simulink library "sm_trackV_lib_chain_underc_i1u2l7"  (R2026a)
settings: Solver=VariableStepAuto
undefined symbols (not defined in the file): Excv, Left, P1, P2, P3, P4, P5, P6, P7, P8, P9, Right
libraries: sm_trackV_lib_chain_underc_elem x26, sm_lib x24, nesl_utility x20, fl_lib x4, sm_trackV_lib_frame_i1u2l7 x2
(part 2 of 2)

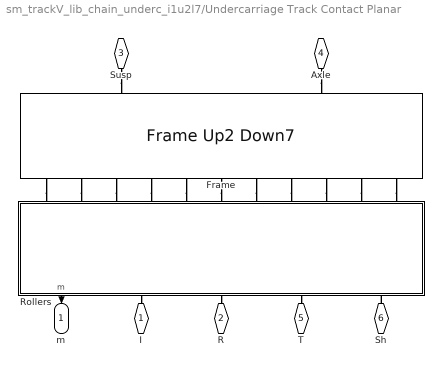
== system sm_trackV_lib_chain_underc_i1u2l7/Undercarriage Track Contact Planar ==
  Frame : sm_trackV_lib_frame_i1u2l7/Frame Up2 Down7  popup_leftOrRight=Right  roller_upper_x=roller_upper_x  roller_lower_x=roller_lower_x  idler_x=idler_x  axle_x=axle_x  roller_upper_y=roller_upper_y  roller_lower_y=roller_lower_y  idler_y=idler_y  axle_y=axle_y  frame_cg_offset=frame_cg_offset  frame_mass=frame_mass  frame_moi=frame_moi  frame_poi=frame_poi  frame_susp_offset=frame_susp_offset
  Rollers : Subsystem  mask(Rollers for Integration with Track Model){sprk_xc=sprk_xc, sprk_len=sprk_len, sprk_rho=sprk_rho, sprk_clr=sprk_clr, sprk_opc=sprk_opc, sprk_contact_geo_ptcld=sprk_contact_geo_ptcld, sprk_contact_geo_rad=sprk_contact_geo_rad, sprk_contact_geo_clr=sprk_contact_geo_clr, sprk_contact_geo_opc=sprk_contact_geo_opc, idler_rad=idler_rad, idler_len=idler_len, idler_rho=idler_rho, idler_clr=idler_clr, idler_opc=idler_opc, idler_contgeo_clr=idler_contgeo_clr, idler_contgeo_opc=idler_contgeo_opc, roller_upper_len=roller_upper_len, roller_upper_rad=roller_upper_rad, roller_upper_rho=roller_upper_rho, roller_upper_clr=roller_upper_clr, roller_upper_opc=roller_upper_opc, roller_upper_contgeo_clr=roller_upper_contgeo_clr, roller_upper_contgeo_opc=roller_upper_contgeo_opc, roller_lower_len=roller_lower_len, roller_lower_rad=roller_lower_rad, roller_lower_rho=roller_lower_rho, roller_lower_clr=roller_lower_clr, roller_lower_opc=roller_lower_opc, roller_lower_contgeo_clr=roller_lower_contgeo_clr, roller_lower_contgeo_opc=roller_lower_contgeo_opc, tensioner_cyl_rad=tensioner_cyl_rad, tensioner_cyl_len=tensioner_cyl_len, tensioner_cyl_rho=tensioner_cyl_rho, tensioner_cyl_clr=tensioner_cyl_clr, tensioner_cyl_opc=tensioner_cyl_opc, tensioner_pist_rad=tensioner_pist_rad, tensioner_pist_len=tensioner_pist_len, tensioner_pist_rho=tensioner_pist_rho, tensioner_pist_clr=tensioner_pist_clr, tensioner_pist_opc=tensioner_pist_opc, tensioner_br_length=tensioner_br_length, tensioner_br_width=tensioner_br_width, tensioner_br_height=tensioner_br_height, tensioner_br_thk=tensioner_br_thk, tensioner_br_rho=tensioner_br_rho, tensioner_br_clr=tensioner_br_clr, tensioner_br_opc=tensioner_br_opc, tensioner_eqpos=tensioner_eqpos, tensioner_x0=tensioner_x0, tensioner_b=tensioner_b, tensioner_k=tensioner_k, popup_sense_roller=Actuator Torque}
      mask prompts: sprk_xc "Extrusion Data [x y] (m)"; sprk_len "Length (m)"; sprk_rho "Density (kg/m^3)"; sprk_clr "Color [R G B] (0-1)"; sprk_opc "Opacity (0-1)"; sprk_contact_geo_ptcld "Point Cloud Data [x y z] (m)"; sprk_contact_geo_rad "Radius (m)"; sprk_contact_geo_clr "Color [R G B] (0-1)"; sprk_contact_geo_opc "Opacity (0-1)"; idler_rad "Radius (m)"; idler_len "Length(m)"; idler_rho "Density (kg/m^3)"; idler_clr "Color [R G B] (0-1)"; idler_opc "Opacity (0-1)"; idler_contgeo_clr "Color [R G B] (0-1)"; idler_contgeo_opc "Opacity (0-1)"; roller_upper_len "Length (m)"; roller_upper_rad "Radius (m)"; roller_upper_rho "Density (kg/m^3)"; roller_upper_clr "Color [R G B] (0-1)"; roller_upper_opc "Opacity (0-1)"; roller_upper_contgeo_clr "Color [R G B] (0-1)"; roller_upper_contgeo_opc "Opacity (0-1)"; roller_lower_len "Length (m)"; roller_lower_rad "Radius (m)"; roller_lower_rho "Density (kg/m^3)"; roller_lower_clr "Color [R G B] (0-1)"; roller_lower_opc "Opacity (0-1)"; roller_lower_contgeo_clr "Color [R G B] (0-1)"; roller_lower_contgeo_opc "Opacity (0-1)"; tensioner_cyl_rad "Radius (m)"; tensioner_cyl_len "Length (m)"; tensioner_cyl_rho "Density (kg/m^3)"; tensioner_cyl_clr "Color [R G B] (0-1)"; tensioner_cyl_opc "Opacity (0-1)"; tensioner_pist_rad "Radius (m)"; tensioner_pist_len "Length (m)"; tensioner_pist_rho "Density (kg/m^3)"; tensioner_pist_clr "Color [R G B] (0-1)"; tensioner_pist_opc "Opacity (0.1)"; tensioner_br_length "Length (m)"; tensioner_br_width "Width (m)"; tensioner_br_height "Height (m)"; tensioner_br_thk "Thickness (m)"; tensioner_br_rho "Density (kg/m^3)"; tensioner_br_clr "Color [R G B] (0-1)"; tensioner_br_opc "Opacity (0.1)"; tensioner_eqpos "Equilibrium Position (m)"; tensioner_x0 "Assembly Position (m)"; tensioner_b "Damping Coefficient (N/(m/s))"; tensioner_k "Stiffness Coefficient (N/m)"; popup_sense_roller "Roller"
      mask help: Models sprocket, rollers, and idler with tensioner. Components have contact geometry for integration with a segmented track model. Contact forces within the track are planar to speed up simulation. The sprocket has a 1D rotational mechanical interface to the drivetrain.
      mask init:
      | % Sensing a constraint force can be computationally expensive
      | % Use popup to turn it off if quantity is not needed
      | bh = gcb;
      | if(strcmp(get_param(bh,'popup_sense_roller'),'Constraint Force'))
      |     SCF = 'on'; STF = 'off';
      |     connectedPort = "fc_out";
      |     senseConstraintTorque = "on";
      |     senseTorqueForce = "off";
      | else
      |     SCF = 'off'; STF = 'on';
      |     connectedPort = "t_out";
      |     senseConstraintTorque = "off";
      |     senseTorqueForce = "on";
      | end
      | 
      | f = Simulink.FindOptions('RegExp',true,'SearchDepth',1);
      | bh_rv = Simulink.findBlocks(bh,...
      |     'Name','Revolute Lower #*',f);
      | bh_ps = Simulink.findBlocks(bh,...
      |     'Name','PS-SL Lower #*',f);
      | [~, indrv] = sort(getfullname(bh_rv));
      | [~, indps] = sort(getfullname(bh_ps));
      | bh_rv = bh_rv(indrv);
      | bh_ps = bh_ps(indps);
      | 
      | bh_rvspr = get_param([bh '/Revolute Sprocket'],'Handle');
      | bh_rvidl = get_param([bh '/Revolute Idler'],'Handle');
      | 
      | bh_psspr = get_param([bh '/PS-SL Sprocket'],'Handle');
      | bh_psidl = get_param([bh '/PS-SL Idler'],'Handle');
      | 
      | bh_rv = [bh_rv; bh_rvidl; bh_rvspr];
      | bh_ps = [bh_ps; bh_psidl; bh_psspr];
      | 
      | for i = 1:length(bh_rv)
      |     port_rv = get_param(bh_rv(i),'PortHandles');
      |     port_ps = get_param(bh_ps(i),'PortHandles');
      |     line_rv = get_param(bh_rv(i),'LineHandles');
      | 
      |     if (i==length(bh_rv))
      |         lineInd = 3; % Sprocket joint senses 2 signals
      |     else
      |         lineInd = 2; % All other joints sense 1 signal
      |     end
      |     delete_line(line_rv.RConn(lineInd))
      | 
      |     set_param(bh_rv(i),'SenseConstraintForce',SCF,'SenseTorqueForce',STF);
      |     simscape.addConnection(bh_rv(i), connectedPort, bh_ps(i),'input');
      | end
      mask TypeOptions sprk_xc: Sprocket/sprk_xc
      mask TypeOptions sprk_len: Sprocket/sprk_len
      mask TypeOptions sprk_rho: Sprocket/sprk_rho
      mask TypeOptions sprk_clr: Sprocket/sprk_clr
      mask TypeOptions sprk_opc: Sprocket/sprk_opc
      mask TypeOptions sprk_contact_geo_ptcld: Sprocket/sprk_contact_geo_ptcld
      mask TypeOptions sprk_contact_geo_rad: Sprocket/sprk_contact_geo_rad
      mask TypeOptions sprk_contact_geo_clr: Sprocket/sprk_contact_geo_clr
      mask TypeOptions sprk_contact_geo_opc: Sprocket/sprk_contact_geo_opc
      mask TypeOptions idler_rad: Idler/idler_rad
      mask TypeOptions idler_len: Idler/idler_len
      mask TypeOptions idler_rho: Idler/idler_rho
      mask TypeOptions idler_clr: Idler/idler_clr
      mask TypeOptions idler_opc: Idler/idler_opc
      mask TypeOptions idler_contgeo_clr: Idler/idler_contgeo_clr
      mask TypeOptions idler_contgeo_opc: Idler/idler_contgeo_opc
      mask TypeOptions roller_upper_len:
      | Roller
      | Upper 1/roller_upper_len | Roller
      | Upper 2/roller_upper_len
      mask TypeOptions roller_upper_rad:
      | Roller
      | Upper 1/roller_upper_rad | Roller
      | Upper 2/roller_upper_rad
      mask TypeOptions roller_upper_rho:
      | Roller
      | Upper 1/roller_upper_rho | Roller
      | Upper 2/roller_upper_rho
      mask TypeOptions roller_upper_clr:
      | Roller
      | Upper 1/roller_upper_clr | Roller
      | Upper 2/roller_upper_clr
      mask TypeOptions roller_upper_opc:
      | Roller
      | Upper 1/roller_upper_opc | Roller
      | Upper 2/roller_upper_opc
      mask TypeOptions roller_upper_contgeo_clr:
      | Roller
      | Upper 1/roller_upper_contgeo_clr | Roller
      | Upper 2/roller_upper_contgeo_clr
      mask TypeOptions roller_upper_contgeo_opc:
      | Roller
      | Upper 1/roller_upper_contgeo_opc | Roller
      | Upper 2/roller_upper_contgeo_opc
      mask TypeOptions roller_lower_len:
      | Roller
      | Lower 1/roller_lower_len | Roller
      | Lower 2/roller_lower_len | Roller
      | Lower 3/roller_lower_len | Roller
      | Lower 4/roller_lower_len | Roller
      | Lower 5/roller_lower_len | Roller
      | Lower 6/roller_lower_len | Roller
      | Lower 7/roller_lower_len
      mask TypeOptions roller_lower_rad:
      | Roller
      | Lower 1/roller_lower_rad | Roller
      | Lower 2/roller_lower_rad | Roller
      | Lower 3/roller_lower_rad | Roller
      | Lower 4/roller_lower_rad | Roller
      | Lower 5/roller_lower_rad | Roller
      | Lower 6/roller_lower_rad | Roller
      | Lower 7/roller_lower_rad
      mask TypeOptions roller_lower_rho:
      | Roller
      | Lower 1/roller_lower_rho | Roller
      | Lower 2/roller_lower_rho | Roller
      | Lower 3/roller_lower_rho | Roller
      | Lower 4/roller_lower_rho | Roller
      | Lower 5/roller_lower_rho | Roller
      | Lower 6/roller_lower_rho | Roller
      | Lower 7/roller_lower_rho
      mask TypeOptions roller_lower_clr:
      | Roller
      | Lower 1/roller_lower_clr | Roller
      | Lower 2/roller_lower_clr | Roller
      | Lower 3/roller_lower_clr | Roller
      | Lower 4/roller_lower_clr | Roller
      | Lower 5/roller_lower_clr | Roller
      | Lower 6/roller_lower_clr | Roller
      | Lower 7/roller_lower_clr
      mask TypeOptions roller_lower_opc:
      | Roller
      | Lower 1/roller_lower_opc | Roller
      | Lower 2/roller_lower_opc | Roller
      | Lower 3/roller_lower_opc | Roller
      | Lower 4/roller_lower_opc | Roller
      | Lower 5/roller_lower_opc | Roller
      | Lower 6/roller_lower_opc | Roller
      | Lower 7/roller_lower_opc
      mask TypeOptions roller_lower_contgeo_clr:
      | Roller
      | Lower 1/roller_lower_contgeo_clr | Roller
      | Lower 2/roller_lower_contgeo_clr | Roller
      | Lower 3/roller_lower_contgeo_clr | Roller
      | Lower 4/roller_lower_contgeo_clr | Roller
      | Lower 5/roller_lower_contgeo_clr | Roller
      | Lower 6/roller_lower_contgeo_clr | Roller
      | Lower 7/roller_lower_contgeo_clr
      mask TypeOptions roller_lower_contgeo_opc:
      | Roller
      | Lower 1/roller_lower_contgeo_opc | Roller
      | Lower 2/roller_lower_contgeo_opc | Roller
      | Lower 3/roller_lower_contgeo_opc | Roller
      | Lower 4/roller_lower_contgeo_opc | Roller
      | Lower 5/roller_lower_contgeo_opc | Roller
      | Lower 6/roller_lower_contgeo_opc | Roller
      | Lower 7/roller_lower_contgeo_opc
      mask TypeOptions tensioner_cyl_rad:
      | Tensioner
      | Cylinder/cyl_rad
      mask TypeOptions tensioner_cyl_len:
      | Tensioner
      | Cylinder/cyl_len
      mask TypeOptions tensioner_cyl_rho:
      | Tensioner
      | Cylinder/cyl_rho
      mask TypeOptions tensioner_cyl_clr:
      | Tensioner
      | Cylinder/cyl_clr
      mask TypeOptions tensioner_cyl_opc:
      | Tensioner
      | Cylinder/cyl_opc
      mask TypeOptions tensioner_pist_rad:
      | Tensioner
      | Piston/pist_rad
      mask TypeOptions tensioner_pist_len:
      | Tensioner
      | Piston/pist_len
      mask TypeOptions tensioner_pist_rho:
      | Tensioner
      | Piston/pist_rho
      mask TypeOptions tensioner_pist_clr:
      | Tensioner
      | Piston/pist_clr
      mask TypeOptions tensioner_pist_opc:
      | Tensioner
      | Piston/pist_opc
      mask TypeOptions tensioner_br_length:
      | Tensioner
      | Piston/br_length
      mask TypeOptions tensioner_br_width:
      | Tensioner
      | Piston/br_width
      mask TypeOptions tensioner_br_height:
      | Tensioner
      | Piston/br_height
      mask TypeOptions tensioner_br_thk:
      | Tensioner
      | Piston/br_thk
      mask TypeOptions tensioner_br_rho:
      | Tensioner
      | Piston/br_rho
      mask TypeOptions tensioner_br_clr:
      | Tensioner
      | Piston/br_clr
      mask TypeOptions tensioner_br_opc:
      | Tensioner
      | Piston/br_opc
      mask TypeOptions tensioner_eqpos:
      | Prismatic
      | Tensioner/EquilibriumPosition
      mask TypeOptions tensioner_x0:
      | Prismatic
      | Tensioner/PositionTargetValue
      mask TypeOptions tensioner_b:
      | Prismatic
      | Tensioner/DampingCoefficient
      mask TypeOptions tensioner_k:
      | Prismatic
      | Tensioner/SpringStiffness
      mask TypeOptions popup_sense_roller: Constraint Force | Actuator Torque
      mask DialogControl cont_sprk Prompt: Sprocket
      mask DialogControl cont_sprk_solid Prompt: Solid
      mask DialogControl cont_sprk_contact_geo Prompt: Contact Geometry
      mask DialogControl cont_idler Prompt: Idler
      mask DialogControl cont_idler_solid Prompt: Solid
      mask DialogControl cont_idler_contact_geo Prompt: Contact Geometry
      mask DialogControl cont_rollers Prompt: Rollers
      mask DialogControl cont_roller_upper Prompt: Upper
      mask DialogControl cont_roller_upper_contact_geo Prompt: Contact Geometry
      mask DialogControl cont_lower Prompt: Lower
      mask DialogControl cont_lower_contact_geo Prompt: Contact Geometry
      mask DialogControl cont_tensioner Prompt: Tensioner
      mask DialogControl cont_tensioner_cyl Prompt: Cylinder
      mask DialogControl cont_tensioner_pist Prompt: Piston
      mask DialogControl cont_tensioner_brkt Prompt: Bracket
      mask DialogControl cont_tensioner_assy Prompt: Assembly
      mask DialogControl cont_sensing Prompt: Sensing
      mask Display:
      | image('sm_excv_track_rollers_IMAGE.png');
      | disp('Pla')
  I : PMIOPort  Side=Right
  R : PMIOPort  Port=2  Side=Right
  Susp : PMIOPort  Port=3  Side=Right
  Axle : PMIOPort  Port=4  Side=Right
  T : PMIOPort  Port=5  Side=Right
  Sh : PMIOPort  Port=6  Side=Right
  m : Outport
  wires:
  Rollers/1(m) -> m/1
  connections:
  Axle/RConn1 -- Frame/LConn2
  Rollers/RConn2 -- R/RConn1
  Susp/RConn1 -- Frame/LConn1
  Rollers/RConn1 -- I/RConn1
  Rollers/RConn3 -- T/RConn1
  Frame/RConn7 -- Rollers/LConn7
  Frame/RConn5 -- Rollers/LConn5
  Frame/RConn4 -- Rollers/LConn4
  Frame/RConn8 -- Rollers/LConn8
  Frame/RConn10 -- Rollers/LConn10
  Frame/RConn9 -- Rollers/LConn9
  Frame/RConn6 -- Rollers/LConn6
  Frame/RConn1 -- Rollers/LConn1
  Frame/RConn11 -- Rollers/LConn11
  Frame/RConn3 -- Rollers/LConn3
  Frame/RConn2 -- Rollers/LConn2
  Sh/RConn1 -- Rollers/RConn4

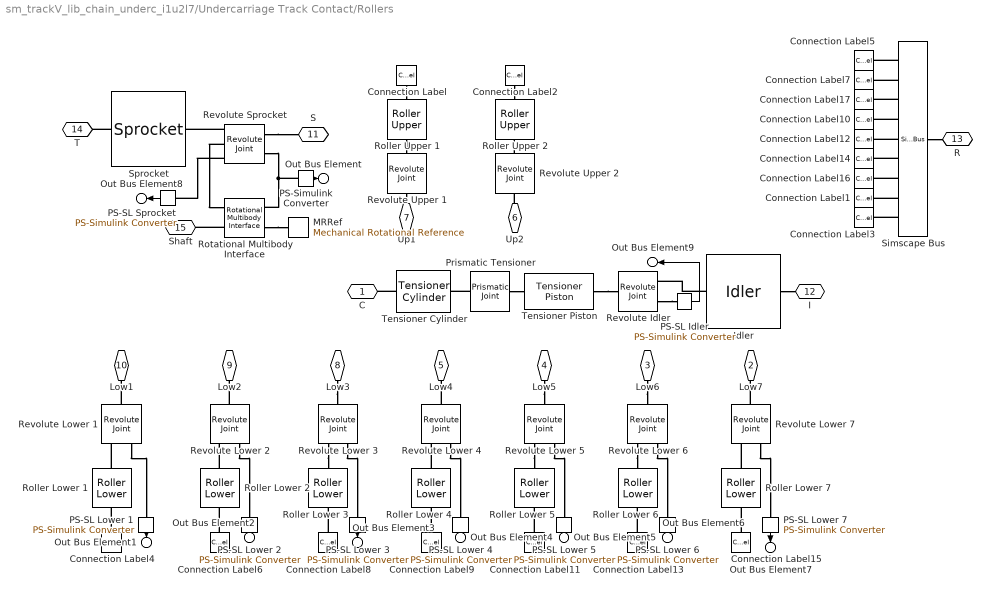
== system sm_trackV_lib_chain_underc_i1u2l7/Undercarriage Track Contact/Rollers ==
  Connection Label : ConnectionLabel  Label=U1
  Connection Label1 : ConnectionLabel  Label=U1
  Connection Label10 : ConnectionLabel  Label=L4
  Connection Label11 : ConnectionLabel  Label=L5
  Connection Label12 : ConnectionLabel  Label=L5
  Connection Label13 : ConnectionLabel  Label=L6
  Connection Label14 : ConnectionLabel  Label=L6
  Connection Label15 : ConnectionLabel  Label=L7
  Connection Label16 : ConnectionLabel  Label=L7
  Connection Label17 : ConnectionLabel  Label=L3
  Connection Label2 : ConnectionLabel  Label=U2
  Connection Label3 : ConnectionLabel  Label=U2
  Connection Label4 : ConnectionLabel  Label=L1
  Connection Label5 : ConnectionLabel  Label=L1
  Connection Label6 : ConnectionLabel  Label=L2
  Connection Label7 : ConnectionLabel  Label=L2
  Connection Label8 : ConnectionLabel  Label=L3
  Connection Label9 : ConnectionLabel  Label=L4
  Idler : sm_trackV_lib_chain_underc_elem/Idler  idler_rad=idler_rad  idler_len=idler_len  idler_rho=idler_rho  idler_clr=idler_clr  idler_opc=idler_opc  idler_contgeo_clr=idler_contgeo_clr  idler_contgeo_opc=idler_contgeo_opc
  MRRef : fl_lib/Mechanical/Rotational Elements/Mechanical Rotational Reference
  PS-SL Idler : nesl_utility/PS-Simulink Converter  PhysicalDomain=network_engine_domain  SubClassName=ps_output  LeftPortType=input  RightPortType=output  PseudoPeriodic=off  Frequencies=[]  VectorFormat=inherit  Unit=inherit  AffineConversion=off
  PS-SL Lower {1..7} (7 alike) : nesl_utility/PS-Simulink Converter  PhysicalDomain=network_engine_domain  SubClassName=ps_output  LeftPortType=input  RightPortType=output  PseudoPeriodic=off  Frequencies=[]  VectorFormat=inherit  Unit=inherit  AffineConversion=off
  PS-SL Sprocket : nesl_utility/PS-Simulink Converter  PhysicalDomain=network_engine_domain  SubClassName=ps_output  LeftPortType=input  RightPortType=output  PseudoPeriodic=off  Frequencies=[]  VectorFormat=inherit  Unit=inherit  AffineConversion=off
  PS-Simulink Converter : nesl_utility/PS-Simulink Converter  PhysicalDomain=network_engine_domain  SubClassName=ps_output  LeftPortType=input  RightPortType=output  PseudoPeriodic=off  Frequencies=[]  VectorFormat=inherit  Unit=inherit  AffineConversion=off
  Prismatic Tensioner : sm_lib/Joints/Prismatic Joint  JointMode=Normal  CompositeWrenchDir=FollowerOnBase  CompositeWrenchFrame=BaseFrame  SenseConstraintForce=off  SenseConstraintTorque=off  SenseTotalForce=off  SenseTotalTorque=off  PositionTargetSpecify=on  PositionTargetPriority=High  PositionTargetValue=tensioner_x0  PositionTargetValueUnits=m  VelocityTargetSpecify=off  VelocityTargetPriority=High  VelocityTargetValue=0  VelocityTargetValueUnits=m/s  EquilibriumPosition=tensioner_eqpos  EquilibriumPositionUnits=m  SpringStiffness=tensioner_k  SpringStiffnessUnits=N/m  DampingCoefficient=tensioner_b  DampingCoefficientUnits=N/(m/s)  LowerLimitSpecify=off  LowerLimitBound=-1  LowerLimitBoundUnits=m  LowerLimitStiffness=1e6  LowerLimitStiffnessUnits=N/m  LowerLimitDamping=1e3  LowerLimitDampingUnits=N/(m/s)  LowerLimitTransitionRegionWidth=1e-4  LowerLimitTransitionRegionWidthUnits=m  UpperLimitSpecify=off  UpperLimitBound=1  UpperLimitBoundUnits=m  UpperLimitStiffness=1e6  UpperLimitStiffnessUnits=N/m  UpperLimitDamping=1e3  UpperLimitDampingUnits=N/(m/s)  UpperLimitTransitionRegionWidth=1e-4  UpperLimitTransitionRegionWidthUnits=m  TorqueActuationMode=NoTorque  MotionActuationMode=ComputedMotion  SensePosition=off  SenseVelocity=off  SenseAcceleration=off  SenseTorqueForce=off  SenseLowerLimitTorqueForce=off  SenseUpperLimitTorqueForce=off
  Revolute Idler : sm_lib/Joints/Revolute Joint  JointMode=Normal  CompositeWrenchDir=FollowerOnBase  CompositeWrenchFrame=BaseFrame  SenseConstraintForce=off  SenseConstraintTorque=off  SenseTotalForce=off  SenseTotalTorque=off  PositionTargetSpecify=off  PositionTargetPriority=Low  PositionTargetValue=0  PositionTargetValueUnits=deg  VelocityTargetSpecify=off  VelocityTargetPriority=High  VelocityTargetValue=0  VelocityTargetValueUnits=deg/s  EquilibriumPosition=0  EquilibriumPositionUnits=rad  SpringStiffness=0  SpringStiffnessUnits=N*m/rad  DampingCoefficient=0  DampingCoefficientUnits=N*m/(rad/s)  LowerLimitSpecify=off  LowerLimitBound=-90  LowerLimitBoundUnits=deg  LowerLimitStiffness=1e4  LowerLimitStiffnessUnits=N*m/deg  LowerLimitDamping=10  LowerLimitDampingUnits=N*m/(deg/s)  LowerLimitTransitionRegionWidth=0.1  LowerLimitTransitionRegionWidthUnits=deg  UpperLimitSpecify=off  UpperLimitBound=90  UpperLimitBoundUnits=deg  UpperLimitStiffness=1e4  UpperLimitStiffnessUnits=N*m/deg  UpperLimitDamping=10  UpperLimitDampingUnits=N*m/(deg/s)  UpperLimitTransitionRegionWidth=0.1  UpperLimitTransitionRegionWidthUnits=deg  TorqueActuationMode=NoTorque  MotionActuationMode=ComputedMotion  SensePosition=off  SenseVelocity=off  SenseAcceleration=off  SenseTorqueForce=on  SenseLowerLimitTorqueForce=off  SenseUpperLimitTorqueForce=off
  Revolute Lower {1..7} (7 alike) : sm_lib/Joints/Revolute Joint  JointMode=Normal  CompositeWrenchDir=FollowerOnBase  CompositeWrenchFrame=BaseFrame  SenseConstraintForce=off  SenseConstraintTorque=off  SenseTotalForce=off  SenseTotalTorque=off  PositionTargetSpecify=off  PositionTargetPriority=Low  PositionTargetValue=0  PositionTargetValueUnits=deg  VelocityTargetSpecify=off  VelocityTargetPriority=High  VelocityTargetValue=0  VelocityTargetValueUnits=deg/s  EquilibriumPosition=0  EquilibriumPositionUnits=rad  SpringStiffness=0  SpringStiffnessUnits=N*m/rad  DampingCoefficient=0  DampingCoefficientUnits=N*m/(rad/s)  LowerLimitSpecify=off  LowerLimitBound=-90  LowerLimitBoundUnits=deg  LowerLimitStiffness=1e4  LowerLimitStiffnessUnits=N*m/deg  LowerLimitDamping=10  LowerLimitDampingUnits=N*m/(deg/s)  LowerLimitTransitionRegionWidth=0.1  LowerLimitTransitionRegionWidthUnits=deg  UpperLimitSpecify=off  UpperLimitBound=90  UpperLimitBoundUnits=deg  UpperLimitStiffness=1e4  UpperLimitStiffnessUnits=N*m/deg  UpperLimitDamping=10  UpperLimitDampingUnits=N*m/(deg/s)  UpperLimitTransitionRegionWidth=0.1  UpperLimitTransitionRegionWidthUnits=deg  TorqueActuationMode=NoTorque  MotionActuationMode=ComputedMotion  SensePosition=off  SenseVelocity=off  SenseAcceleration=off  SenseTorqueForce=on  SenseLowerLimitTorqueForce=off  SenseUpperLimitTorqueForce=off
  Revolute Sprocket : sm_lib/Joints/Revolute Joint  JointMode=Normal  CompositeWrenchDir=FollowerOnBase  CompositeWrenchFrame=BaseFrame  SenseConstraintForce=off  SenseConstraintTorque=off  SenseTotalForce=off  SenseTotalTorque=off  PositionTargetSpecify=off  PositionTargetPriority=Low  PositionTargetValue=0  PositionTargetValueUnits=deg  VelocityTargetSpecify=off  VelocityTargetPriority=High  VelocityTargetValue=0  VelocityTargetValueUnits=deg/s  EquilibriumPosition=0  EquilibriumPositionUnits=rad  SpringStiffness=0  SpringStiffnessUnits=N*m/rad  DampingCoefficient=0  DampingCoefficientUnits=N*m/(rad/s)  LowerLimitSpecify=off  LowerLimitBound=-90  LowerLimitBoundUnits=deg  LowerLimitStiffness=1e4  LowerLimitStiffnessUnits=N*m/deg  LowerLimitDamping=10  LowerLimitDampingUnits=N*m/(deg/s)  LowerLimitTransitionRegionWidth=0.1  LowerLimitTransitionRegionWidthUnits=deg  UpperLimitSpecify=off  UpperLimitBound=90  UpperLimitBoundUnits=deg  UpperLimitStiffness=1e4  UpperLimitStiffnessUnits=N*m/deg  UpperLimitDamping=10  UpperLimitDampingUnits=N*m/(deg/s)  UpperLimitTransitionRegionWidth=0.1  UpperLimitTransitionRegionWidthUnits=deg  TorqueActuationMode=InputTorque  MotionActuationMode=ComputedMotion  SensePosition=off  SenseVelocity=on  SenseAcceleration=off  SenseTorqueForce=on  SenseLowerLimitTorqueForce=off  SenseUpperLimitTorqueForce=off
  Revolute Upper 1 : sm_lib/Joints/Revolute Joint  JointMode=Normal  CompositeWrenchDir=FollowerOnBase  CompositeWrenchFrame=BaseFrame  SenseConstraintForce=off  SenseConstraintTorque=off  SenseTotalForce=off  SenseTotalTorque=off  PositionTargetSpecify=off  PositionTargetPriority=Low  PositionTargetValue=0  PositionTargetValueUnits=deg  VelocityTargetSpecify=off  VelocityTargetPriority=High  VelocityTargetValue=0  VelocityTargetValueUnits=deg/s  EquilibriumPosition=0  EquilibriumPositionUnits=rad  SpringStiffness=0  SpringStiffnessUnits=N*m/rad  DampingCoefficient=0  DampingCoefficientUnits=N*m/(rad/s)  LowerLimitSpecify=off  LowerLimitBound=-90  LowerLimitBoundUnits=deg  LowerLimitStiffness=1e4  LowerLimitStiffnessUnits=N*m/deg  LowerLimitDamping=10  LowerLimitDampingUnits=N*m/(deg/s)  LowerLimitTransitionRegionWidth=0.1  LowerLimitTransitionRegionWidthUnits=deg  UpperLimitSpecify=off  UpperLimitBound=90  UpperLimitBoundUnits=deg  UpperLimitStiffness=1e4  UpperLimitStiffnessUnits=N*m/deg  UpperLimitDamping=10  UpperLimitDampingUnits=N*m/(deg/s)  UpperLimitTransitionRegionWidth=0.1  UpperLimitTransitionRegionWidthUnits=deg  TorqueActuationMode=NoTorque  MotionActuationMode=ComputedMotion  SensePosition=off  SenseVelocity=off  SenseAcceleration=off  SenseTorqueForce=off  SenseLowerLimitTorqueForce=off  SenseUpperLimitTorqueForce=off
  Revolute Upper 2 : sm_lib/Joints/Revolute Joint  JointMode=Normal  CompositeWrenchDir=FollowerOnBase  CompositeWrenchFrame=BaseFrame  SenseConstraintForce=off  SenseConstraintTorque=off  SenseTotalForce=off  SenseTotalTorque=off  PositionTargetSpecify=off  PositionTargetPriority=Low  PositionTargetValue=0  PositionTargetValueUnits=deg  VelocityTargetSpecify=off  VelocityTargetPriority=High  VelocityTargetValue=0  VelocityTargetValueUnits=deg/s  EquilibriumPosition=0  EquilibriumPositionUnits=rad  SpringStiffness=0  SpringStiffnessUnits=N*m/rad  DampingCoefficient=0  DampingCoefficientUnits=N*m/(rad/s)  LowerLimitSpecify=off  LowerLimitBound=-90  LowerLimitBoundUnits=deg  LowerLimitStiffness=1e4  LowerLimitStiffnessUnits=N*m/deg  LowerLimitDamping=10  LowerLimitDampingUnits=N*m/(deg/s)  LowerLimitTransitionRegionWidth=0.1  LowerLimitTransitionRegionWidthUnits=deg  UpperLimitSpecify=off  UpperLimitBound=90  UpperLimitBoundUnits=deg  UpperLimitStiffness=1e4  UpperLimitStiffnessUnits=N*m/deg  UpperLimitDamping=10  UpperLimitDampingUnits=N*m/(deg/s)  UpperLimitTransitionRegionWidth=0.1  UpperLimitTransitionRegionWidthUnits=deg  TorqueActuationMode=NoTorque  MotionActuationMode=ComputedMotion  SensePosition=off  SenseVelocity=off  SenseAcceleration=off  SenseTorqueForce=off  SenseLowerLimitTorqueForce=off  SenseUpperLimitTorqueForce=off
  Roller Lower {1..7} (7 alike) : sm_trackV_lib_chain_underc_elem/Roller Lower  roller_lower_rad=roller_lower_rad  roller_lower_len=roller_lower_len  roller_lower_rho=roller_lower_rho  roller_lower_clr=roller_lower_clr  roller_lower_opc=roller_lower_opc  roller_lower_contgeo_clr=roller_lower_contgeo_clr  roller_lower_contgeo_opc=roller_lower_contgeo_opc
      settings: LibrarySourceBlock=sm_chain_drive_lib/Pulley_Bot
  Roller Upper 1 : sm_trackV_lib_chain_underc_elem/Roller Upper  roller_upper_rad=roller_upper_rad  roller_upper_len=roller_upper_len  roller_upper_rho=roller_upper_rho  roller_upper_clr=roller_upper_clr  roller_upper_opc=roller_upper_opc  roller_upper_contgeo_clr=roller_upper_contgeo_clr  roller_upper_contgeo_opc=roller_upper_contgeo_opc
      settings: LibrarySourceBlock=sm_chain_drive_lib/Pulley_Top
  Roller Upper 2 : sm_trackV_lib_chain_underc_elem/Roller Upper  roller_upper_rad=roller_upper_rad  roller_upper_len=roller_upper_len  roller_upper_rho=roller_upper_rho  roller_upper_clr=roller_upper_clr  roller_upper_opc=roller_upper_opc  roller_upper_contgeo_clr=roller_upper_contgeo_clr  roller_upper_contgeo_opc=roller_upper_contgeo_opc
      settings: LibrarySourceBlock=sm_chain_drive_lib/Pulley_Top
  Rotational Multibody Interface : fl_lib/Mechanical/Multibody Interfaces/Rotational Multibody Interface
  Simscape Bus : SimscapeBus  HierarchyStrings=P1;P2;P3;P4;P5;P6;P7;P8;P9  ConnectionType=Bus: CBO_Roller9
  Sprocket : sm_trackV_lib_chain_underc_elem/Sprocket  sprk_xc=sprk_xc  sprk_len=sprk_len  sprk_rho=sprk_rho  sprk_clr=sprk_clr  sprk_opc=sprk_opc  sprk_contact_geo_ptcld=sprk_contact_geo_ptcld  sprk_contact_geo_rad=sprk_contact_geo_rad  sprk_contact_geo_clr=sprk_contact_geo_clr  sprk_contact_geo_opc=sprk_contact_geo_opc
  Tensioner Cylinder : sm_trackV_lib_chain_underc_elem/Tensioner Cylinder  cyl_rad=tensioner_cyl_rad  cyl_len=tensioner_cyl_len  cyl_rho=tensioner_cyl_rho  cyl_clr=tensioner_cyl_clr  cyl_opc=tensioner_cyl_opc  brk_len=Excv.Idler.Tensioner.bracket.len  brk_thk=Excv.Idler.Tensioner.bracket.thk  pist_len=Excv.Idler.Tensioner.piston.len
      settings: LibrarySourceBlock=sm_chain_drive_lib/Idler_Housing
  Tensioner Piston : sm_trackV_lib_chain_underc_elem/Tensioner Piston  pist_rad=tensioner_pist_rad  pist_len=tensioner_pist_len  pist_rho=tensioner_pist_rho  pist_clr=tensioner_pist_clr  pist_opc=tensioner_pist_opc  br_height=tensioner_br_height  br_length=tensioner_br_length  br_width=tensioner_br_width  br_rho=tensioner_br_rho  br_thk=tensioner_br_thk  br_clr=tensioner_br_clr  br_opc=tensioner_br_opc
      settings: LibrarySourceBlock=sm_chain_drive_lib/ldler_Damper
  C : PMIOPort  Side=Left
  Low7 : PMIOPort  Port=2  Side=Left
  Low6 : PMIOPort  Port=3  Side=Left
  Low5 : PMIOPort  Port=4  Side=Left
  Low4 : PMIOPort  Port=5  Side=Left
  Up2 : PMIOPort  Port=6  Side=Left
  Up1 : PMIOPort  Port=7  Side=Left
  Low3 : PMIOPort  Port=8  Side=Left
  Low2 : PMIOPort  Port=9  Side=Left
  Low1 : PMIOPort  Port=10  Side=Left
  S : PMIOPort  Port=11  Side=Left
  I : PMIOPort  Port=12  Side=Right
  R : PMIOPort  Port=13  Side=Right
  T : PMIOPort  Port=14  Side=Right
  Shaft : PMIOPort  Port=15  Side=Right
  Out Bus Element : Outport  PortName=m  Element=tSprk
  Out Bus Element1 : Outport  PortName=m  Element=RL1
  Out Bus Element2 : Outport  PortName=m  Element=RL2
  Out Bus Element3 : Outport  PortName=m  Element=RL3
  Out Bus Element4 : Outport  PortName=m  Element=RL4
  Out Bus Element5 : Outport  PortName=m  Element=RL5
  Out Bus Element6 : Outport  PortName=m  Element=RL6
  Out Bus Element7 : Outport  PortName=m  Element=RL7
  Out Bus Element8 : Outport  PortName=m  Element=XSprk
  Out Bus Element9 : Outport  PortName=m  Element=XIdlerF
  wires:
  PS-Simulink Converter/1 -> Out Bus Element/1
  PS-SL Lower 1/1 -> Out Bus Element1/1
  PS-SL Lower 2/1 -> Out Bus Element2/1
  PS-SL Lower 3/1 -> Out Bus Element3/1
  PS-SL Lower 4/1 -> Out Bus Element4/1
  PS-SL Lower 5/1 -> Out Bus Element5/1
  PS-SL Lower 6/1 -> Out Bus Element6/1
  PS-SL Lower 7/1 -> Out Bus Element7/1
  PS-SL Sprocket/1 -> Out Bus Element8/1
  PS-SL Idler/1 -> Out Bus Element9/1
  connections:
  Idler/RConn1 -- I/RConn1
  Connection Label13/LConn1 -- Roller Lower 6/RConn1
  Connection Label6/LConn1 -- Roller Lower 2/RConn1
  Connection Label/LConn1 -- Roller Upper 1/RConn1
  Revolute Upper 1/LConn1 -- Up1/RConn1
  Connection Label9/LConn1 -- Roller Lower 4/RConn1
  Connection Label15/LConn1 -- Roller Lower 7/RConn1
  Revolute Lower 6/RConn1 -- Roller Lower 6/LConn1
  Connection Label8/LConn1 -- Roller Lower 3/RConn1
  Revolute Sprocket/LConn1 -- S/RConn1
  Connection Label11/LConn1 -- Roller Lower 5/RConn1
  Simscape Bus/RConn1 -- R/RConn1
  Idler/LConn1 -- Revolute Idler/RConn1
  Revolute Sprocket/RConn1 -- Sprocket/LConn1
  Prismatic Tensioner/LConn1 -- Tensioner Cylinder/RConn1
  Revolute Lower 5/RConn1 -- Roller Lower 5/LConn1
  Revolute Upper 2/RConn1 -- Roller Upper 2/LConn1
  Revolute Lower 2/LConn1 -- Low2/RConn1
  Tensioner Piston/RConn1 -- Revolute Idler/LConn1
  Sprocket/RConn1 -- T/RConn1
  Connection Label4/LConn1 -- Roller Lower 1/RConn1
  Revolute Lower 4/LConn1 -- Low4/RConn1
  Revolute Lower 3/RConn1 -- Roller Lower 3/LConn1
  Revolute Lower 7/LConn1 -- Low7/RConn1
  Revolute Lower 1/LConn1 -- Low1/RConn1
  Connection Label2/LConn1 -- Roller Upper 2/RConn1
  Simscape Bus/LConn9 -- Connection Label3/LConn1
  Simscape Bus/LConn8 -- Connection Label1/LConn1
  Simscape Bus/LConn4 -- Connection Label10/LConn1
  Simscape Bus/LConn3 -- Connection Label17/LConn1
  Simscape Bus/LConn2 -- Connection Label7/LConn1
  Simscape Bus/LConn7 -- Connection Label16/LConn1
  Simscape Bus/LConn6 -- Connection Label14/LConn1
  Simscape Bus/LConn5 -- Connection Label12/LConn1
  Simscape Bus/LConn1 -- Connection Label5/LConn1
  Tensioner Cylinder/LConn1 -- C/RConn1
  Prismatic Tensioner/RConn1 -- Tensioner Piston/LConn1
  Low5/RConn1 -- Revolute Lower 5/LConn1
  Roller Lower 2/LConn1 -- Revolute Lower 2/RConn1
  Low3/RConn1 -- Revolute Lower 3/LConn1
  Roller Lower 7/LConn1 -- Revolute Lower 7/RConn1
  Roller Lower 1/LConn1 -- Revolute Lower 1/RConn1
  Roller Lower 4/LConn1 -- Revolute Lower 4/RConn1
  Low6/RConn1 -- Revolute Lower 6/LConn1
  Roller Upper 1/LConn1 -- Revolute Upper 1/RConn1
  Up2/RConn1 -- Revolute Upper 2/LConn1
  Revolute Sprocket/LConn2 -- Rotational Multibody Interface/LConn1 -- PS-Simulink Converter/LConn1
  Rotational Multibody Interface/RConn2 -- Shaft/RConn1
  Rotational Multibody Interface/LConn2 -- MRRef/LConn1
  Revolute Sprocket/RConn2 -- Rotational Multibody Interface/RConn1
  Revolute Lower 1/RConn2 -- PS-SL Lower 1/LConn1
  Revolute Lower 2/RConn2 -- PS-SL Lower 2/LConn1
  Revolute Lower 3/RConn2 -- PS-SL Lower 3/LConn1
  Revolute Lower 4/RConn2 -- PS-SL Lower 4/LConn1
  Revolute Lower 5/RConn2 -- PS-SL Lower 5/LConn1
  Revolute Lower 6/RConn2 -- PS-SL Lower 6/LConn1
  Revolute Lower 7/RConn2 -- PS-SL Lower 7/LConn1
  Revolute Idler/RConn2 -- PS-SL Idler/LConn1
  Revolute Sprocket/RConn3 -- PS-SL Sprocket/LConn1

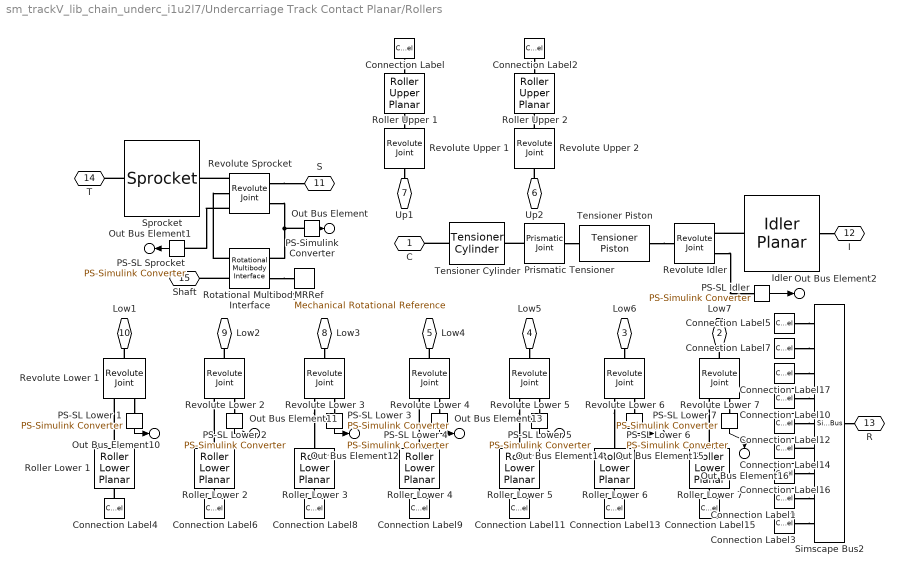
== system sm_trackV_lib_chain_underc_i1u2l7/Undercarriage Track Contact Planar/Rollers ==
  Connection Label : ConnectionLabel  Label=U1
  Connection Label1 : ConnectionLabel  Label=U1
  Connection Label10 : ConnectionLabel  Label=L4
  Connection Label11 : ConnectionLabel  Label=L5
  Connection Label12 : ConnectionLabel  Label=L5
  Connection Label13 : ConnectionLabel  Label=L6
  Connection Label14 : ConnectionLabel  Label=L6
  Connection Label15 : ConnectionLabel  Label=L7
  Connection Label16 : ConnectionLabel  Label=L7
  Connection Label17 : ConnectionLabel  Label=L3
  Connection Label2 : ConnectionLabel  Label=U2
  Connection Label3 : ConnectionLabel  Label=U2
  Connection Label4 : ConnectionLabel  Label=L1
  Connection Label5 : ConnectionLabel  Label=L1
  Connection Label6 : ConnectionLabel  Label=L2
  Connection Label7 : ConnectionLabel  Label=L2
  Connection Label8 : ConnectionLabel  Label=L3
  Connection Label9 : ConnectionLabel  Label=L4
  Idler : sm_trackV_lib_chain_underc_elem/Idler Planar  idler_rad=idler_rad  idler_len=idler_len  idler_rho=idler_rho  idler_clr=idler_clr  idler_opc=idler_opc  idler_contgeo_clr=idler_contgeo_clr  idler_contgeo_opc=idler_contgeo_opc
  MRRef : fl_lib/Mechanical/Rotational Elements/Mechanical Rotational Reference
  PS-SL Idler : nesl_utility/PS-Simulink Converter  PhysicalDomain=network_engine_domain  SubClassName=ps_output  LeftPortType=input  RightPortType=output  PseudoPeriodic=off  Frequencies=[]  VectorFormat=inherit  Unit=inherit  AffineConversion=off
  PS-SL Lower {1..7} (7 alike) : nesl_utility/PS-Simulink Converter  PhysicalDomain=network_engine_domain  SubClassName=ps_output  LeftPortType=input  RightPortType=output  PseudoPeriodic=off  Frequencies=[]  VectorFormat=inherit  Unit=inherit  AffineConversion=off
  PS-SL Sprocket : nesl_utility/PS-Simulink Converter  PhysicalDomain=network_engine_domain  SubClassName=ps_output  LeftPortType=input  RightPortType=output  PseudoPeriodic=off  Frequencies=[]  VectorFormat=inherit  Unit=inherit  AffineConversion=off
  PS-Simulink Converter : nesl_utility/PS-Simulink Converter  PhysicalDomain=network_engine_domain  SubClassName=ps_output  LeftPortType=input  RightPortType=output  PseudoPeriodic=off  Frequencies=[]  VectorFormat=inherit  Unit=inherit  AffineConversion=off
  Prismatic Tensioner : sm_lib/Joints/Prismatic Joint  JointMode=Normal  CompositeWrenchDir=FollowerOnBase  CompositeWrenchFrame=BaseFrame  SenseConstraintForce=off  SenseConstraintTorque=off  SenseTotalForce=off  SenseTotalTorque=off  PositionTargetSpecify=on  PositionTargetPriority=High  PositionTargetValue=tensioner_x0  PositionTargetValueUnits=m  VelocityTargetSpecify=off  VelocityTargetPriority=High  VelocityTargetValue=0  VelocityTargetValueUnits=m/s  EquilibriumPosition=tensioner_eqpos  EquilibriumPositionUnits=m  SpringStiffness=tensioner_k  SpringStiffnessUnits=N/m  DampingCoefficient=tensioner_b  DampingCoefficientUnits=N/(m/s)  LowerLimitSpecify=off  LowerLimitBound=-1  LowerLimitBoundUnits=m  LowerLimitStiffness=1e6  LowerLimitStiffnessUnits=N/m  LowerLimitDamping=1e3  LowerLimitDampingUnits=N/(m/s)  LowerLimitTransitionRegionWidth=1e-4  LowerLimitTransitionRegionWidthUnits=m  UpperLimitSpecify=off  UpperLimitBound=1  UpperLimitBoundUnits=m  UpperLimitStiffness=1e6  UpperLimitStiffnessUnits=N/m  UpperLimitDamping=1e3  UpperLimitDampingUnits=N/(m/s)  UpperLimitTransitionRegionWidth=1e-4  UpperLimitTransitionRegionWidthUnits=m  TorqueActuationMode=NoTorque  MotionActuationMode=ComputedMotion  SensePosition=off  SenseVelocity=off  SenseAcceleration=off  SenseTorqueForce=off  SenseLowerLimitTorqueForce=off  SenseUpperLimitTorqueForce=off
  Revolute Idler : sm_lib/Joints/Revolute Joint  JointMode=Normal  CompositeWrenchDir=FollowerOnBase  CompositeWrenchFrame=BaseFrame  SenseConstraintForce=off  SenseConstraintTorque=off  SenseTotalForce=off  SenseTotalTorque=off  PositionTargetSpecify=off  PositionTargetPriority=Low  PositionTargetValue=0  PositionTargetValueUnits=deg  VelocityTargetSpecify=off  VelocityTargetPriority=High  VelocityTargetValue=0  VelocityTargetValueUnits=deg/s  EquilibriumPosition=0  EquilibriumPositionUnits=rad  SpringStiffness=0  SpringStiffnessUnits=N*m/rad  DampingCoefficient=0  DampingCoefficientUnits=N*m/(rad/s)  LowerLimitSpecify=off  LowerLimitBound=-90  LowerLimitBoundUnits=deg  LowerLimitStiffness=1e4  LowerLimitStiffnessUnits=N*m/deg  LowerLimitDamping=10  LowerLimitDampingUnits=N*m/(deg/s)  LowerLimitTransitionRegionWidth=0.1  LowerLimitTransitionRegionWidthUnits=deg  UpperLimitSpecify=off  UpperLimitBound=90  UpperLimitBoundUnits=deg  UpperLimitStiffness=1e4  UpperLimitStiffnessUnits=N*m/deg  UpperLimitDamping=10  UpperLimitDampingUnits=N*m/(deg/s)  UpperLimitTransitionRegionWidth=0.1  UpperLimitTransitionRegionWidthUnits=deg  TorqueActuationMode=NoTorque  MotionActuationMode=ComputedMotion  SensePosition=off  SenseVelocity=off  SenseAcceleration=off  SenseTorqueForce=on  SenseLowerLimitTorqueForce=off  SenseUpperLimitTorqueForce=off
  Revolute Lower {1..7} (7 alike) : sm_lib/Joints/Revolute Joint  JointMode=Normal  CompositeWrenchDir=FollowerOnBase  CompositeWrenchFrame=BaseFrame  SenseConstraintForce=off  SenseConstraintTorque=off  SenseTotalForce=off  SenseTotalTorque=off  PositionTargetSpecify=off  PositionTargetPriority=Low  PositionTargetValue=0  PositionTargetValueUnits=deg  VelocityTargetSpecify=off  VelocityTargetPriority=High  VelocityTargetValue=0  VelocityTargetValueUnits=deg/s  EquilibriumPosition=0  EquilibriumPositionUnits=rad  SpringStiffness=0  SpringStiffnessUnits=N*m/rad  DampingCoefficient=0  DampingCoefficientUnits=N*m/(rad/s)  LowerLimitSpecify=off  LowerLimitBound=-90  LowerLimitBoundUnits=deg  LowerLimitStiffness=1e4  LowerLimitStiffnessUnits=N*m/deg  LowerLimitDamping=10  LowerLimitDampingUnits=N*m/(deg/s)  LowerLimitTransitionRegionWidth=0.1  LowerLimitTransitionRegionWidthUnits=deg  UpperLimitSpecify=off  UpperLimitBound=90  UpperLimitBoundUnits=deg  UpperLimitStiffness=1e4  UpperLimitStiffnessUnits=N*m/deg  UpperLimitDamping=10  UpperLimitDampingUnits=N*m/(deg/s)  UpperLimitTransitionRegionWidth=0.1  UpperLimitTransitionRegionWidthUnits=deg  TorqueActuationMode=NoTorque  MotionActuationMode=ComputedMotion  SensePosition=off  SenseVelocity=off  SenseAcceleration=off  SenseTorqueForce=on  SenseLowerLimitTorqueForce=off  SenseUpperLimitTorqueForce=off
  Revolute Sprocket : sm_lib/Joints/Revolute Joint  JointMode=Normal  CompositeWrenchDir=FollowerOnBase  CompositeWrenchFrame=BaseFrame  SenseConstraintForce=off  SenseConstraintTorque=off  SenseTotalForce=off  SenseTotalTorque=off  PositionTargetSpecify=off  PositionTargetPriority=Low  PositionTargetValue=0  PositionTargetValueUnits=deg  VelocityTargetSpecify=off  VelocityTargetPriority=High  VelocityTargetValue=0  VelocityTargetValueUnits=deg/s  EquilibriumPosition=0  EquilibriumPositionUnits=rad  SpringStiffness=0  SpringStiffnessUnits=N*m/rad  DampingCoefficient=0  DampingCoefficientUnits=N*m/(rad/s)  LowerLimitSpecify=off  LowerLimitBound=-90  LowerLimitBoundUnits=deg  LowerLimitStiffness=1e4  LowerLimitStiffnessUnits=N*m/deg  LowerLimitDamping=10  LowerLimitDampingUnits=N*m/(deg/s)  LowerLimitTransitionRegionWidth=0.1  LowerLimitTransitionRegionWidthUnits=deg  UpperLimitSpecify=off  UpperLimitBound=90  UpperLimitBoundUnits=deg  UpperLimitStiffness=1e4  UpperLimitStiffnessUnits=N*m/deg  UpperLimitDamping=10  UpperLimitDampingUnits=N*m/(deg/s)  UpperLimitTransitionRegionWidth=0.1  UpperLimitTransitionRegionWidthUnits=deg  TorqueActuationMode=InputTorque  MotionActuationMode=ComputedMotion  SensePosition=off  SenseVelocity=on  SenseAcceleration=off  SenseTorqueForce=on  SenseLowerLimitTorqueForce=off  SenseUpperLimitTorqueForce=off
  Revolute Upper 1 : sm_lib/Joints/Revolute Joint  JointMode=Normal  CompositeWrenchDir=FollowerOnBase  CompositeWrenchFrame=BaseFrame  SenseConstraintForce=off  SenseConstraintTorque=off  SenseTotalForce=off  SenseTotalTorque=off  PositionTargetSpecify=off  PositionTargetPriority=Low  PositionTargetValue=0  PositionTargetValueUnits=deg  VelocityTargetSpecify=off  VelocityTargetPriority=High  VelocityTargetValue=0  VelocityTargetValueUnits=deg/s  EquilibriumPosition=0  EquilibriumPositionUnits=rad  SpringStiffness=0  SpringStiffnessUnits=N*m/rad  DampingCoefficient=0  DampingCoefficientUnits=N*m/(rad/s)  LowerLimitSpecify=off  LowerLimitBound=-90  LowerLimitBoundUnits=deg  LowerLimitStiffness=1e4  LowerLimitStiffnessUnits=N*m/deg  LowerLimitDamping=10  LowerLimitDampingUnits=N*m/(deg/s)  LowerLimitTransitionRegionWidth=0.1  LowerLimitTransitionRegionWidthUnits=deg  UpperLimitSpecify=off  UpperLimitBound=90  UpperLimitBoundUnits=deg  UpperLimitStiffness=1e4  UpperLimitStiffnessUnits=N*m/deg  UpperLimitDamping=10  UpperLimitDampingUnits=N*m/(deg/s)  UpperLimitTransitionRegionWidth=0.1  UpperLimitTransitionRegionWidthUnits=deg  TorqueActuationMode=NoTorque  MotionActuationMode=ComputedMotion  SensePosition=off  SenseVelocity=off  SenseAcceleration=off  SenseTorqueForce=off  SenseLowerLimitTorqueForce=off  SenseUpperLimitTorqueForce=off
  Revolute Upper 2 : sm_lib/Joints/Revolute Joint  JointMode=Normal  CompositeWrenchDir=FollowerOnBase  CompositeWrenchFrame=BaseFrame  SenseConstraintForce=off  SenseConstraintTorque=off  SenseTotalForce=off  SenseTotalTorque=off  PositionTargetSpecify=off  PositionTargetPriority=Low  PositionTargetValue=0  PositionTargetValueUnits=deg  VelocityTargetSpecify=off  VelocityTargetPriority=High  VelocityTargetValue=0  VelocityTargetValueUnits=deg/s  EquilibriumPosition=0  EquilibriumPositionUnits=rad  SpringStiffness=0  SpringStiffnessUnits=N*m/rad  DampingCoefficient=0  DampingCoefficientUnits=N*m/(rad/s)  LowerLimitSpecify=off  LowerLimitBound=-90  LowerLimitBoundUnits=deg  LowerLimitStiffness=1e4  LowerLimitStiffnessUnits=N*m/deg  LowerLimitDamping=10  LowerLimitDampingUnits=N*m/(deg/s)  LowerLimitTransitionRegionWidth=0.1  LowerLimitTransitionRegionWidthUnits=deg  UpperLimitSpecify=off  UpperLimitBound=90  UpperLimitBoundUnits=deg  UpperLimitStiffness=1e4  UpperLimitStiffnessUnits=N*m/deg  UpperLimitDamping=10  UpperLimitDampingUnits=N*m/(deg/s)  UpperLimitTransitionRegionWidth=0.1  UpperLimitTransitionRegionWidthUnits=deg  TorqueActuationMode=NoTorque  MotionActuationMode=ComputedMotion  SensePosition=off  SenseVelocity=off  SenseAcceleration=off  SenseTorqueForce=off  SenseLowerLimitTorqueForce=off  SenseUpperLimitTorqueForce=off
  Roller Lower {1..7} (7 alike) : sm_trackV_lib_chain_underc_elem/Roller Lower Planar  roller_lower_rad=roller_lower_rad  roller_lower_len=roller_lower_len  roller_lower_rho=roller_lower_rho  roller_lower_clr=roller_lower_clr  roller_lower_opc=roller_lower_opc  roller_lower_contgeo_clr=roller_lower_contgeo_clr  roller_lower_contgeo_opc=roller_lower_contgeo_opc
  Roller Upper 1 : sm_trackV_lib_chain_underc_elem/Roller Upper Planar  roller_upper_rad=roller_upper_rad  roller_upper_len=roller_upper_len  roller_upper_rho=roller_upper_rho  roller_upper_clr=roller_upper_clr  roller_upper_opc=roller_upper_opc  roller_upper_contgeo_clr=roller_upper_contgeo_clr  roller_upper_contgeo_opc=roller_upper_contgeo_opc
  Roller Upper 2 : sm_trackV_lib_chain_underc_elem/Roller Upper Planar  roller_upper_rad=roller_upper_rad  roller_upper_len=roller_upper_len  roller_upper_rho=roller_upper_rho  roller_upper_clr=roller_upper_clr  roller_upper_opc=roller_upper_opc  roller_upper_contgeo_clr=roller_upper_contgeo_clr  roller_upper_contgeo_opc=roller_upper_contgeo_opc
  Rotational Multibody Interface : fl_lib/Mechanical/Multibody Interfaces/Rotational Multibody Interface
  Simscape Bus2 : SimscapeBus  HierarchyStrings=P1;P2;P3;P4;P5;P6;P7;P8;P9  ConnectionType=Bus: CBO_Roller9
  Sprocket : sm_trackV_lib_chain_underc_elem/Sprocket  sprk_xc=sprk_xc  sprk_len=sprk_len  sprk_rho=sprk_rho  sprk_clr=sprk_clr  sprk_opc=sprk_opc  sprk_contact_geo_ptcld=sprk_contact_geo_ptcld  sprk_contact_geo_rad=sprk_contact_geo_rad  sprk_contact_geo_clr=sprk_contact_geo_clr  sprk_contact_geo_opc=sprk_contact_geo_opc
  Tensioner Cylinder : sm_trackV_lib_chain_underc_elem/Tensioner Cylinder  cyl_rad=tensioner_cyl_rad  cyl_len=tensioner_cyl_len  cyl_rho=tensioner_cyl_rho  cyl_clr=tensioner_cyl_clr  cyl_opc=tensioner_cyl_opc  brk_len=Excv.Idler.Tensioner.bracket.len  brk_thk=Excv.Idler.Tensioner.bracket.thk  pist_len=Excv.Idler.Tensioner.piston.len
      settings: LibrarySourceBlock=sm_chain_drive_lib/Idler_Housing
  Tensioner Piston : sm_trackV_lib_chain_underc_elem/Tensioner Piston  pist_rad=tensioner_pist_rad  pist_len=tensioner_pist_len  pist_rho=tensioner_pist_rho  pist_clr=tensioner_pist_clr  pist_opc=tensioner_pist_opc  br_height=tensioner_br_height  br_length=tensioner_br_length  br_width=tensioner_br_width  br_rho=tensioner_br_rho  br_thk=tensioner_br_thk  br_clr=tensioner_br_clr  br_opc=tensioner_br_opc
      settings: LibrarySourceBlock=sm_chain_drive_lib/ldler_Damper
  C : PMIOPort  Side=Left
  Low7 : PMIOPort  Port=2  Side=Left
  Low6 : PMIOPort  Port=3  Side=Left
  Low5 : PMIOPort  Port=4  Side=Left
  Low4 : PMIOPort  Port=5  Side=Left
  Up2 : PMIOPort  Port=6  Side=Left
  Up1 : PMIOPort  Port=7  Side=Left
  Low3 : PMIOPort  Port=8  Side=Left
  Low2 : PMIOPort  Port=9  Side=Left
  Low1 : PMIOPort  Port=10  Side=Left
  S : PMIOPort  Port=11  Side=Left
  I : PMIOPort  Port=12  Side=Right
  R : PMIOPort  Port=13  Side=Right
  T : PMIOPort  Port=14  Side=Right
  Shaft : PMIOPort  Port=15  Side=Right
  Out Bus Element : Outport  PortName=m  Element=tSprk
  Out Bus Element10 : Outport  PortName=m  Element=RL1
  Out Bus Element11 : Outport  PortName=m  Element=RL2
  Out Bus Element12 : Outport  PortName=m  Element=RL3
  Out Bus Element13 : Outport  PortName=m  Element=RL4
  Out Bus Element14 : Outport  PortName=m  Element=RL5
  Out Bus Element15 : Outport  PortName=m  Element=RL6
  Out Bus Element16 : Outport  PortName=m  Element=RL7
  Out Bus Element1 : Outport  PortName=m  Element=XSprk
  Out Bus Element2 : Outport  PortName=m  Element=XIdlerF
  wires:
  PS-SL Lower 6/1 -> Out Bus Element15/1
  PS-SL Lower 1/1 -> Out Bus Element10/1
  PS-SL Lower 4/1 -> Out Bus Element13/1
  PS-SL Lower 5/1 -> Out Bus Element14/1
  PS-SL Lower 3/1 -> Out Bus Element12/1
  PS-SL Lower 7/1 -> Out Bus Element16/1
  PS-SL Lower 2/1 -> Out Bus Element11/1
  PS-Simulink Converter/1 -> Out Bus Element/1
  PS-SL Sprocket/1 -> Out Bus Element1/1
  PS-SL Idler/1 -> Out Bus Element2/1
  connections:
  Idler/RConn1 -- I/RConn1
  Connection Label13/LConn1 -- Roller Lower 6/RConn1
  Connection Label6/LConn1 -- Roller Lower 2/RConn1
  Connection Label/LConn1 -- Roller Upper 1/RConn1
  Revolute Upper 1/LConn1 -- Up1/RConn1
  Connection Label9/LConn1 -- Roller Lower 4/RConn1
  Connection Label15/LConn1 -- Roller Lower 7/RConn1
  Revolute Lower 6/RConn1 -- Roller Lower 6/LConn1
  Connection Label8/LConn1 -- Roller Lower 3/RConn1
  Revolute Sprocket/LConn1 -- S/RConn1
  Connection Label11/LConn1 -- Roller Lower 5/RConn1
  Simscape Bus2/RConn1 -- R/RConn1
  Idler/LConn1 -- Revolute Idler/RConn1
  Revolute Sprocket/RConn1 -- Sprocket/LConn1
  Prismatic Tensioner/LConn1 -- Tensioner Cylinder/RConn1
  Revolute Lower 5/RConn1 -- Roller Lower 5/LConn1
  Revolute Upper 2/RConn1 -- Roller Upper 2/LConn1
  Revolute Lower 2/LConn1 -- Low2/RConn1
  Tensioner Piston/RConn1 -- Revolute Idler/LConn1
  Sprocket/RConn1 -- T/RConn1
  Connection Label4/LConn1 -- Roller Lower 1/RConn1
  Revolute Lower 4/LConn1 -- Low4/RConn1
  Revolute Lower 3/RConn1 -- Roller Lower 3/LConn1
  Revolute Lower 7/LConn1 -- Low7/RConn1
  Revolute Lower 1/LConn1 -- Low1/RConn1
  Connection Label2/LConn1 -- Roller Upper 2/RConn1
  Connection Label3/LConn1 -- Simscape Bus2/LConn9
  Connection Label1/LConn1 -- Simscape Bus2/LConn8
  Connection Label10/LConn1 -- Simscape Bus2/LConn4
  Connection Label17/LConn1 -- Simscape Bus2/LConn3
  Connection Label7/LConn1 -- Simscape Bus2/LConn2
  Connection Label16/LConn1 -- Simscape Bus2/LConn7
  Simscape Bus2/LConn6 -- Connection Label14/LConn1
  Connection Label12/LConn1 -- Simscape Bus2/LConn5
  Connection Label5/LConn1 -- Simscape Bus2/LConn1
  Tensioner Cylinder/LConn1 -- C/RConn1
  Prismatic Tensioner/RConn1 -- Tensioner Piston/LConn1
  Low5/RConn1 -- Revolute Lower 5/LConn1
  Roller Lower 2/LConn1 -- Revolute Lower 2/RConn1
  Low3/RConn1 -- Revolute Lower 3/LConn1
  Roller Lower 7/LConn1 -- Revolute Lower 7/RConn1
  Roller Lower 1/LConn1 -- Revolute Lower 1/RConn1
  Roller Lower 4/LConn1 -- Revolute Lower 4/RConn1
  Low6/RConn1 -- Revolute Lower 6/LConn1
  Roller Upper 1/LConn1 -- Revolute Upper 1/RConn1
  Up2/RConn1 -- Revolute Upper 2/LConn1
  Revolute Sprocket/LConn2 -- Rotational Multibody Interface/LConn1 -- PS-Simulink Converter/LConn1
  Rotational Multibody Interface/RConn1 -- Revolute Sprocket/RConn2
  Rotational Multibody Interface/RConn2 -- Shaft/RConn1
  Rotational Multibody Interface/LConn2 -- MRRef/LConn1
  Revolute Lower 1/RConn2 -- PS-SL Lower 1/LConn1
  Revolute Lower 2/RConn2 -- PS-SL Lower 2/LConn1
  Revolute Lower 3/RConn2 -- PS-SL Lower 3/LConn1
  Revolute Lower 4/RConn2 -- PS-SL Lower 4/LConn1
  Revolute Lower 5/RConn2 -- PS-SL Lower 5/LConn1
  Revolute Lower 6/RConn2 -- PS-SL Lower 6/LConn1
  Revolute Lower 7/RConn2 -- PS-SL Lower 7/LConn1
  Revolute Idler/RConn2 -- PS-SL Idler/LConn1
  Revolute Sprocket/RConn3 -- PS-SL Sprocket/LConn1
